simulink model "Boost_con_panel"  (R2017b)
settings: Solver=FixedStepAuto  StartTime=0.0  StopTime=100e-3  FixedStep=125e-9  RelTol=1e-3
settings Model: Creator=rodoo  LastModifiedBy=rodoo

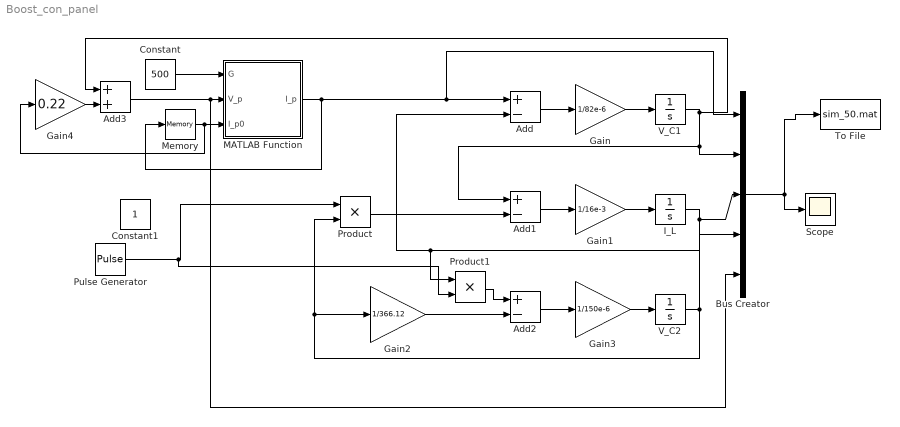
== system Boost_con_panel ==
  Add : Sum  Inputs=+-
  Add1 : Sum  Inputs=+-
  Add2 : Sum  Inputs=+-
  Add3 : Sum
  Bus Creator : BusCreator  Inputs=5
  Constant : Constant  Value=500
  Constant1 : Constant
  Gain : Gain  Gain=1/82e-6
  Gain1 : Gain  Gain=1/16e-3
  Gain2 : Gain  Gain=1/366.12
  Gain3 : Gain  Gain=1/150e-6
  Gain4 : Gain  Gain=0.22
  I_L : Integrator  LimitOutput=on  LowerSaturationLimit=0
  MATLAB Function : MATLAB Function  TreatAsAtomicUnit=on
  Memory : Memory
  Product : Product
  Product1 : Product
  Pulse Generator : DiscretePulseGenerator  PulseType=Time based  Period=20e-6  PulseWidth=50  VectorParams1D=off
  Scope : Scope
  To File : ToFile  Filename=sim_50.mat
  V_C1 : Integrator  LimitOutput=on  LowerSaturationLimit=-9.563
  V_C2 : Integrator  LimitOutput=on  LowerSaturationLimit=0
  wires:
  Memory/1 -> Gain4/1, MATLAB Function/3(I_p0)
  MATLAB Function/1(I_p) -> Bus Creator/1, Add/1, Memory/1
  I_L/1 -> Product1/1, Add/2, Bus Creator/3
  V_C2/1 -> Product/2, Gain2/1, Bus Creator/4
  Gain/1 -> V_C1/1
  Add/1 -> Gain/1
  Gain1/1 -> I_L/1
  Add1/1 -> Gain1/1
  Gain2/1 -> Add2/2
  Gain3/1 -> V_C2/1
  Add2/1 -> Gain3/1
  V_C1/1 -> Add3/1, Bus Creator/2, Add1/1
  Constant/1 -> MATLAB Function/1(G)
  Bus Creator/1 -> Scope/1, To File/1
  Add3/1 -> Bus Creator/5, MATLAB Function/2(V_p)
  Gain4/1 -> Add3/2
  Product/1 -> Add1/2
  Product1/1 -> Add2/1
  Pulse Generator/1 -> Product1/2, Product/1

== matlab function Boost_con_panel/MATLAB Function ==
  data: G input; I_p output; V_p input; I_p0 input
function I_p = panel(G,V_p,I_p0)
   N_s=420;
    
    G_nom=1000;
    I_sc0=9.04004;
    I_o=3.1944118e-8;
   V_t=3.21157239e-2;
    R_s=4.4167825e-3;
    R_sh=1000;
    V_p1=V_p/N_s;
    
    f=(I_sc0*G/G_nom)-(I_o*(exp((V_p1+I_p0*R_s)/V_t)-1))-((V_p1+I_p0*R_s)/R_sh)-I_p0;
    df=-(I_o*R_s/V_t)*exp((V_p1+I_p0*R_s)/V_t)-(R_s/R_sh)-1;
    I_p=I_p0-(f/df);
    
    error = abs(I_p0-I_p);

    while error > 0.00001
        I_p0 = I_p;
        f=(I_sc0*G/G_nom)-(I_o*(exp((V_p1+I_p0*R_s)/V_t)-1))-((V_p1+I_p0*R_s)/R_sh)-I_p0;
        df=-(I_o*R_s/V_t)*exp((V_p1+I_p0*R_s)/V_t)-(R_s/R_sh)-1;
        I_p=I_p0-(f/df);
         
        error = abs(I_p0-I_p);
    end;
    if I_p < 0
        I_p = 0;
    end;
end
